simulink model "Skydiver"  (R2025b)
settings: Solver=VariableStepAuto  StartTime=0.0  StopTime=30  RelTol=1e-3
undefined symbols (not defined in the file): Air, Ao, CD, g, m
settings Model: Creator=Samuel  LastModifiedBy=Samuel

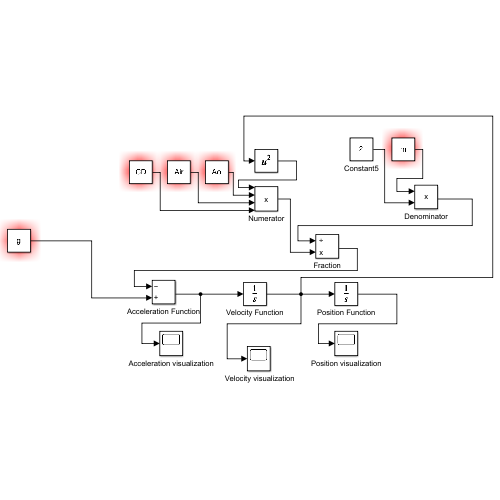
[thumbnail: Simulink's stored preview of the top-level diagram]
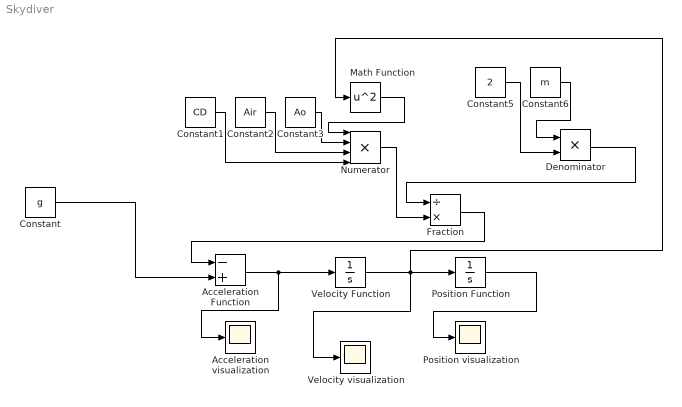
== system Skydiver ==
  " Velocity visualization" : Scope
      settings: AxesScalingNumUpdates=100  ActiveDisplayYMinimum=-18.88422627917226  ActiveDisplayYMaximum=72.286848962734183
  Acceleration Function : Sum  Inputs=-+
  Acceleration visualization : Scope
      settings: ActiveDisplayYMinimum=-1.596852107849144  ActiveDisplayYMaximum=11.262789625016502  DataLoggingVariableName=ScopeData2
  Constant : Constant  Value=g
  Constant1 : Constant  Value=CD
  Constant2 : Constant  Value=Air
  Constant3 : Constant  Value=Ao
  Constant5 : Constant  Value=2
  Constant6 : Constant  Value=m
  Denominator : Product
  Fraction : Product  Inputs=/*
  Math Function : Math  Operator=square
  Numerator : Product  Inputs=4
  Position Function : Integrator
  Position visualization : Scope
      settings: ActiveDisplayYMinimum=-684.97025361558758  ActiveDisplayYMaximum=1998.3313588991855
  Velocity Function : Integrator
  wires:
  Constant1/1 -> Numerator/4
  Constant2/1 -> Numerator/3
  Constant3/1 -> Numerator/2
  Math Function/1 -> Numerator/1
  Constant5/1 -> Denominator/2
  Constant6/1 -> Denominator/1
  Numerator/1 -> Fraction/2
  Denominator/1 -> Fraction/1
  Constant/1 -> Acceleration Function/2
  Fraction/1 -> Acceleration Function/1
  Acceleration Function/1 -> Acceleration visualization/1, Velocity Function/1
  Position Function/1 -> Position visualization/1
  Velocity Function/1 -> Math Function/1, Position Function/1, " Velocity visualization"/1
